simulink model "DGL2_03"  (R2018a)
settings: Solver=VariableStepAuto  StartTime=0.0  StopTime=10.0  RelTol=1e-3
values from neighbouring files (symbols this model uses):
  C = [1, 0, 0, 0 ... (first row only)    [bldc_motor.m]    (also in test_simulink.m = 1)
  Tau = La/Ra    (= 0.00267462686567)    [test_DC_Motor.m]    (also in test_simulink.m = 10319.9174407; ueb_simulink_ofen.m = 10319.9174407)
  u_in = 1    [test_simulink.m]
  w_2 = 1/(L*C)    (= 1)    [test_simulink.m]
undefined symbols (not defined in the file or in its folder): a, b
settings Model: Creator=Horst  LastModifiedBy=Horst

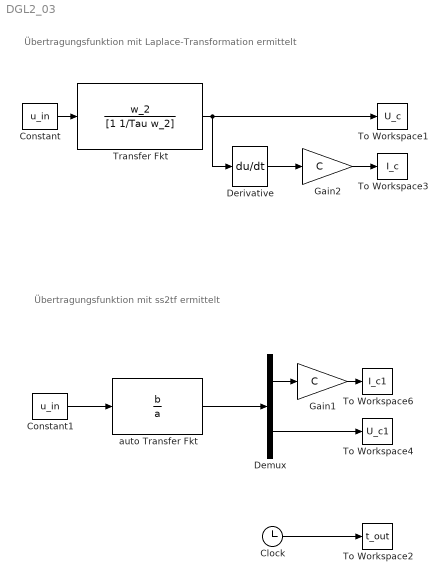
== system DGL2_03 ==
  note: Übertragungsfunktion mit Laplace-Transformation ermittelt
  note: Übertragungsfunktion mit ss2tf ermittelt
  Clock : Clock
  Constant : Constant  Value=u_in
  Constant1 : Constant  Value=u_in
  Demux : Demux  Outputs=2
  Derivative : Derivative
  Gain1 : Gain  Gain=C
  Gain2 : Gain  Gain=C
  To Workspace1 : ToWorkspace  VariableName=U_c  SampleTime=-1
  To Workspace2 : ToWorkspace  VariableName=t_out  SampleTime=-1
  To Workspace3 : ToWorkspace  VariableName=I_c  SampleTime=-1
  To Workspace4 : ToWorkspace  VariableName=U_c1  SampleTime=-1
  To Workspace6 : ToWorkspace  VariableName=I_c1  SampleTime=-1
  Transfer Fkt : TransferFcn  Numerator=w_2  Denominator=[1 1/Tau w_2]
  auto Transfer Fkt : TransferFcn  Numerator=b  Denominator=a
  wires:
  Clock/1 -> To Workspace2/1
  Constant/1 -> Transfer Fkt/1
  Transfer Fkt/1 -> Derivative/1, To Workspace1/1
  Derivative/1 -> Gain2/1
  Gain2/1 -> To Workspace3/1
  Constant1/1 -> auto Transfer Fkt/1
  Demux/2 -> To Workspace4/1
  auto Transfer Fkt/1 -> Demux/1
  Demux/1 -> Gain1/1
  Gain1/1 -> To Workspace6/1
